simulink model "surge"  (R2015a)
settings: Solver=ode45  StartTime=0.0  StopTime=10.0  RelTol=1e-3
settings Model: Creator=JRG94  LastModifiedBy=JRG94

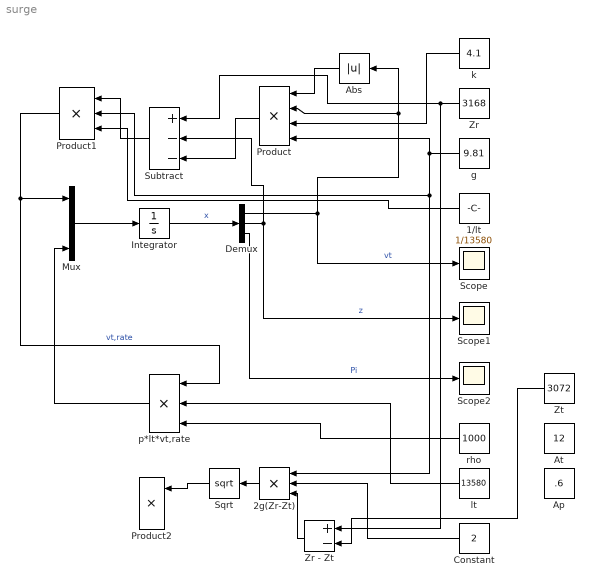
== system surge ==
  1/lt : Constant  Value=1/13580
  2g(Zr-Zt) : Product  Inputs=3
  Abs : Abs
  Ap : Constant  Value=.6
  At : Constant  Value=12
  Constant : Constant  Value=2
  Demux : Demux  Outputs=3
  Integrator : Integrator
  Mux : Mux  Inputs=3
  Product : Product  Inputs=4
  Product1 : Product  Inputs=3
  Product2 : Product  Inputs=3
  Scope : Scope
  Scope1 : Scope
  Scope2 : Scope
      settings: SaveName=ScopeData2
  Sqrt : Sqrt  SaturateOnIntegerOverflow=on
  Subtract : Sum  Inputs=+--
  Zr : Constant  Value=3168
  Zr - Zt : Sum  Inputs=+-
  Zt : Constant  Value=3072
  g : Constant  Value=9.81
  k : Constant  Value=4.1
  lt : Constant  Value=13580
  p*lt*vt,rate : Product  Inputs=3
  rho : Constant  Value=1000
  wires:
  Mux/1 -> Integrator/1
  Integrator/1 -> Demux/1  "x"
  Demux/1 -> Product/2, Abs/1, Scope/1  "vt"
  Demux/2 -> Scope1/1, Subtract/2  "z"
  Demux/3 -> Scope2/1  "Pi"
  Abs/1 -> Product/1
  k/1 -> Product/3
  Zr/1 -> Zr - Zt/1, Subtract/1
  Product/1 -> Subtract/3
  Subtract/1 -> Product1/1
  g/1 -> 2g(Zr-Zt)/1, Product1/2, Product/4
  1/lt/1 -> Product1/3
  Product1/1 -> p*lt*vt,rate/1, Mux/1  "vt,rate"
  p*lt*vt,rate/1 -> Mux/3
  rho/1 -> p*lt*vt,rate/3
  lt/1 -> p*lt*vt,rate/2
  Constant/1 -> 2g(Zr-Zt)/2
  Zt/1 -> Zr - Zt/2
  Zr - Zt/1 -> 2g(Zr-Zt)/3
  2g(Zr-Zt)/1 -> Sqrt/1
  Sqrt/1 -> Product2/1
